simulink model "SIMULATION FILE"  (R2023b)
settings: Solver=VariableStepAuto  StartTime=0.0  StopTime=2.5  RelTol=1e-3
InitFcn:
  | Rs1=0.22;
  | Rsh1=100000;
  | Voc1=0.7;
  | Isc1=0.04;
  | 
  | Rs2=0.22;
  | Rsh2=360;
  | Voc2=0.7;
  | Isc2=0.04;
  | 
  | ki=0.00005926;
  | %ki=0;
  | q=1.6e-19;
  | K=1.30e-23;
  | n=1.3;
  | Ego=1.1;
  | Tn=298;
  | Ns=1;
libraries: simulink x2
settings Model: Creator=smdm6  LastModifiedBy=yasaswini

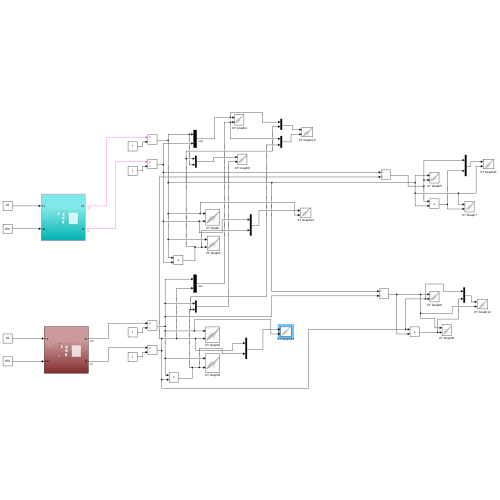
[thumbnail: Simulink's stored preview of the top-level diagram]
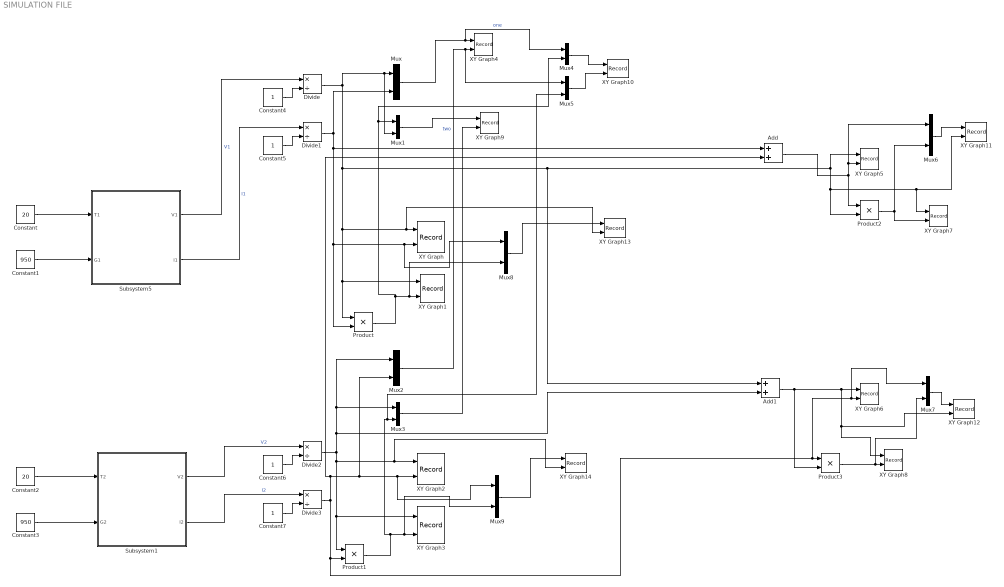
== system SIMULATION FILE ==
  Add : Sum
  Add1 : Sum
  Constant : Constant  Value=20
  Constant1 : Constant  Value=950
  Constant2 : Constant  Value=20
  Constant3 : Constant  Value=950
  Constant{4..7} (4 alike) : Constant
  Divide{,1..3} (4 alike) : Product  Inputs=*/
  Mux{,1..9} (10 alike) : Mux  Inputs=2
  Product{,1..3} (4 alike) : Product
  Subsystem1 : Subsystem
  Subsystem5 : Subsystem
  XY Graph : Record  FileSettingsInternal="{\"entries\":[{\"content\":{\"excelSettings\":{\"content\":{},\"type\":\"Streamout.ExcelSettings\"}},\"type\":\"Streamout.FileSettingStorage\",\"uuid\":\"\"}],\"packageUris\":[\"http:\\/\\/schema.mathworks.com\\/mf0\\/streamout_blocks\\/R2020a\"],\"version\":\"1.0\"}"  Layout=[1 1]  SignalsInternal="{\"entries\":[{\"content\":{\"signals\":[{\"content\":{\"blockPath\":[],\"dimensions\":[1],\"domain\":\"\",\"lineColor\":\"#edb120\",\"port\":1,\"sid\":[\"\"],\"signalID\":1,\"signalName\":\"Divide\"},\"type\":\"RecordBlkView.Signal\",\"uuid\":\"\"},{\"content\":{\"blockPath\":[],\"dimensions\":[1],\"domain\":\"\",\"lineColor\":\"#7e2f8e\",\"port\":2,\"sid\":[\"\"],\"signalID\":2,\"signalName\":\"Divide1\"},\"type\":\"RecordBlkView.Signal\",\"uuid\":\"\"}]},\"type\":\"RecordBlkView.InputSignals\",\"uuid\":\"\"}],\"packageUris\":[\"http:\\/\\/schema.mathworks.com\\/mf0\\/streamout_blocks\\/R2020a\"],\"version\":\"1.0\"}"  VisualizationBindings="{\"xyplotplugin\":{\"info\":[{\"series\":[],\"subplotID\":1}]}}"  CompatibilityTag=XY  st=-1
  XY Graph1 : Record  FileSettingsInternal="{\"entries\":[{\"content\":{\"excelSettings\":{\"content\":{},\"type\":\"Streamout.ExcelSettings\"}},\"type\":\"Streamout.FileSettingStorage\",\"uuid\":\"\"}],\"packageUris\":[\"http:\\/\\/schema.mathworks.com\\/mf0\\/streamout_blocks\\/R2020a\"],\"version\":\"1.0\"}"  Layout=[1 1]  SignalsInternal="{\"entries\":[{\"content\":{\"signals\":[{\"content\":{\"blockPath\":[],\"dimensions\":[1],\"domain\":\"\",\"lineColor\":\"#77ac30\",\"port\":1,\"sid\":[\"\"],\"signalID\":1,\"signalName\":\"Divide\"},\"type\":\"RecordBlkView.Signal\",\"uuid\":\"\"},{\"content\":{\"blockPath\":[],\"dimensions\":[1],\"domain\":\"\",\"lineColor\":\"#4dbeee\",\"port\":2,\"sid\":[\"\"],\"signalID\":2,\"signalName\":\"Product\"},\"type\":\"RecordBlkView.Signal\",\"uuid\":\"\"}]},\"type\":\"RecordBlkView.InputSignals\",\"uuid\":\"\"}],\"packageUris\":[\"http:\\/\\/schema.mathworks.com\\/mf0\\/streamout_blocks\\/R2020a\"],\"version\":\"1.0\"}"  VisualizationBindings="{\"xyplotplugin\":{\"info\":[{\"series\":[],\"subplotID\":1}]}}"  CompatibilityTag=XY  st=-1
  XY Graph10 : Record  FileSettingsInternal="{\"entries\":[{\"content\":{\"excelSettings\":{\"content\":{},\"type\":\"Streamout.ExcelSettings\"}},\"type\":\"Streamout.FileSettingStorage\",\"uuid\":\"\"}],\"packageUris\":[\"http:\\/\\/schema.mathworks.com\\/mf0\\/streamout_blocks\\/R2020a\"],\"version\":\"1.0\"}"  Layout=[1 1]  SignalsInternal="{\"entries\":[{\"content\":{\"signals\":[{\"content\":{\"blockPath\":[],\"dimensions\":[3],\"domain\":\"\",\"hasChildren\":true,\"lineColor\":\"#a2142f\",\"port\":1,\"sid\":[\"\"],\"signalID\":1,\"signalName\":\"Mux4\"},\"type\":\"RecordBlkView.Signal\",\"uuid\":\"\"},{\"content\":{\"blockPath\":[],\"channel\":[1],\"dimensions\":[3],\"domain\":\"\",\"lineColor\":\"#139fff\",\"parentID\":1,\"port\":1,\"sid\":[\"\"],\"signalID\":2,\"signalName\":\"Mux4\"},\"type\":\"RecordBlkView.Signal\",\"uuid\":\"\"},{\"content\":{\"blockPath\":[],\"dimensions\":[3],\"domain\":\"\",\"hasChildren\":true,\"lineColor\":\"#ff6929\",\"port\":2,\"sid\":[\"\"],\"signalID\":3,\"signalName\":\"Mux5\"},\"type\":\"RecordBlkView.Signal\",\"uuid\":\"\"},{\"content\":{\"blockPath\":[],\"channel\":[1],\"dimensions\":[3],\"domain\":\"\",\"lineColor\":\"#b746ff\",\"parentID\":3,\"port\":2,\"sid\":[\"\"],\"signalID\":4,\"signalName\":\"Mux5\"},\"type\":\"RecordBlkView.Signal\",\"uuid\":\"\"},{\"content\":{\"blockPath\":[],\"channel\":[2],\"dimensions\":[3],\"domain\":\"\",\"lineColor\":\"#0072bd\",\"parentID\":1,\"port\":1,\"sid\":[\"\"],\"signalID\":5,\"signalName\":\"Mux4\"},\"type\":\"RecordBlkView.Signal\",\"uuid\":\"\"},{\"content\":{\"blockPath\":[],\"channel\":[3],\"dimensions\":[3],\"domain\":\"\",\"lineColor\":\"#d95319\",\"parentID\":1,\"port\":1,\"sid\":[\"\"],\"signalID\":6,\"signalName\":\"Mux4\"},\"type\":\"RecordBlkView.Signal\",\"uuid\":\"\"},{\"content\":{\"blockPath\":[],\"channel\":[2],\"dimensions\":[3],\"domain\":\"\",\"lineColor\":\"#edb120\",\"parentID\":3,\"port\":2,\"sid\":[\"\"],\"signalID\":7,\"signalName\":\"Mux5\"},\"type\":\"RecordBlkView.Signal\",\"uuid\":\"\"},{\"content\":{\"blockPath\":[],\"channel\":[3],\"dimensions\":[3],\"domain\":\"\",\"lineColor\":\"#7e2f8e\",\"parentID\":3,\"port\":2,\"sid\":[\"\"],\"signalID\":8,\"signalName\":\"Mux5\"},\"type\":\"RecordBlkView.Signal\",\"uuid\":\"\"}]},\"type\":\"RecordBlkView.InputSignals\",\"uuid\":\"\"}],\"packageUris\":[\"http:\\/\\/schema.mathworks.com\\/mf0\\/streamout_blocks\\/R2020a\"],\"version\":\"1.0\"}"  VisualizationBindings="{\"xyplotplugin\":{\"info\":[{\"series\":[],\"subplotID\":1}]}}"  CompatibilityTag=XY
  XY Graph11 : Record  FileSettingsInternal="{\"entries\":[{\"content\":{\"excelSettings\":{\"content\":{},\"type\":\"Streamout.ExcelSettings\"}},\"type\":\"Streamout.FileSettingStorage\",\"uuid\":\"\"}],\"packageUris\":[\"http:\\/\\/schema.mathworks.com\\/mf0\\/streamout_blocks\\/R2020a\"],\"version\":\"1.0\"}"  Layout=[1 1]  SignalsInternal="{\"entries\":[{\"content\":{\"signals\":[{\"content\":{\"blockPath\":[],\"dimensions\":[2],\"domain\":\"\",\"hasChildren\":true,\"lineColor\":\"#64d413\",\"port\":1,\"sid\":[\"\"],\"signalID\":1,\"signalName\":\"Mux6\"},\"type\":\"RecordBlkView.Signal\",\"uuid\":\"\"},{\"content\":{\"blockPath\":[],\"channel\":[1],\"dimensions\":[2],\"domain\":\"\",\"lineColor\":\"#ff13a6\",\"parentID\":1,\"port\":1,\"sid\":[\"\"],\"signalID\":2,\"signalName\":\"Mux6\"},\"type\":\"RecordBlkView.Signal\",\"uuid\":\"\"},{\"content\":{\"blockPath\":[],\"dimensions\":[1],\"domain\":\"\",\"lineColor\":\"#fe330a\",\"port\":2,\"sid\":[\"\"],\"signalID\":3,\"signalName\":\"Divide\"},\"type\":\"RecordBlkView.Signal\",\"uuid\":\"\"},{\"content\":{\"blockPath\":[],\"channel\":[2],\"dimensions\":[2],\"domain\":\"\",\"lineColor\":\"#77ac30\",\"parentID\":1,\"port\":1,\"sid\":[\"\"],\"signalID\":4,\"signalName\":\"Mux6\"},\"type\":\"RecordBlkView.Signal\",\"uuid\":\"\"}]},\"type\":\"RecordBlkView.InputSignals\",\"uuid\":\"\"}],\"packageUris\":[\"http:\\/\\/schema.mathworks.com\\/mf0\\/streamout_blocks\\/R2020a\"],\"version\":\"1.0\"}"  VisualizationBindings="{\"xyplotplugin\":{\"info\":[{\"series\":[],\"subplotID\":1}]}}"  CompatibilityTag=XY
  XY Graph12 : Record  FileSettingsInternal="{\"entries\":[{\"content\":{\"excelSettings\":{\"content\":{},\"type\":\"Streamout.ExcelSettings\"}},\"type\":\"Streamout.FileSettingStorage\",\"uuid\":\"\"}],\"packageUris\":[\"http:\\/\\/schema.mathworks.com\\/mf0\\/streamout_blocks\\/R2020a\"],\"version\":\"1.0\"}"  Layout=[1 1]  SignalsInternal="{\"entries\":[{\"content\":{\"signals\":[{\"content\":{\"blockPath\":[],\"dimensions\":[2],\"domain\":\"\",\"hasChildren\":true,\"lineColor\":\"#22b573\",\"port\":1,\"sid\":[\"\"],\"signalID\":1,\"signalName\":\"Mux7\"},\"type\":\"RecordBlkView.Signal\",\"uuid\":\"\"},{\"content\":{\"blockPath\":[],\"channel\":[1],\"dimensions\":[2],\"domain\":\"\",\"lineColor\":\"#0072bd\",\"parentID\":1,\"port\":1,\"sid\":[\"\"],\"signalID\":2,\"signalName\":\"Mux7\"},\"type\":\"RecordBlkView.Signal\",\"uuid\":\"\"},{\"content\":{\"blockPath\":[],\"dimensions\":[1],\"domain\":\"\",\"lineColor\":\"#d95319\",\"port\":2,\"sid\":[\"\"],\"signalID\":3,\"signalName\":\"Add1\"},\"type\":\"RecordBlkView.Signal\",\"uuid\":\"\"},{\"content\":{\"blockPath\":[],\"channel\":[2],\"dimensions\":[2],\"domain\":\"\",\"lineColor\":\"#4dbeee\",\"parentID\":1,\"port\":1,\"sid\":[\"\"],\"signalID\":4,\"signalName\":\"Mux7\"},\"type\":\"RecordBlkView.Signal\",\"uuid\":\"\"}]},\"type\":\"RecordBlkView.InputSignals\",\"uuid\":\"\"}],\"packageUris\":[\"http:\\/\\/schema.mathworks.com\\/mf0\\/streamout_blocks\\/R2020a\"],\"version\":\"1.0\"}"  VisualizationBindings="{\"xyplotplugin\":{\"info\":[{\"series\":[],\"subplotID\":1}]}}"  CompatibilityTag=XY
  XY Graph13 : Record  FileSettingsInternal="{\"entries\":[{\"content\":{\"excelSettings\":{\"content\":{},\"type\":\"Streamout.ExcelSettings\"}},\"type\":\"Streamout.FileSettingStorage\",\"uuid\":\"\"}],\"packageUris\":[\"http:\\/\\/schema.mathworks.com\\/mf0\\/streamout_blocks\\/R2020a\"],\"version\":\"1.0\"}"  Layout=[1 1]  SignalsInternal="{\"entries\":[{\"content\":{\"signals\":[{\"content\":{\"blockPath\":[],\"dimensions\":[2],\"domain\":\"\",\"hasChildren\":true,\"lineColor\":\"#edb120\",\"port\":1,\"sid\":[\"\"],\"signalID\":1,\"signalName\":\"Mux8\"},\"type\":\"RecordBlkView.Signal\",\"uuid\":\"\"},{\"content\":{\"blockPath\":[],\"channel\":[1],\"dimensions\":[2],\"domain\":\"\",\"lineColor\":\"#7e2f8e\",\"parentID\":1,\"port\":1,\"sid\":[\"\"],\"signalID\":2,\"signalName\":\"Mux8\"},\"type\":\"RecordBlkView.Signal\",\"uuid\":\"\"},{\"content\":{\"blockPath\":[],\"dimensions\":[1],\"domain\":\"\",\"lineColor\":\"#77ac30\",\"port\":2,\"sid\":[\"\"],\"signalID\":3,\"signalName\":\"Divide\"},\"type\":\"RecordBlkView.Signal\",\"uuid\":\"\"},{\"content\":{\"blockPath\":[],\"channel\":[2],\"dimensions\":[2],\"domain\":\"\",\"lineColor\":\"#a2142f\",\"parentID\":1,\"port\":1,\"sid\":[\"\"],\"signalID\":4,\"signalName\":\"Mux8\"},\"type\":\"RecordBlkView.Signal\",\"uuid\":\"\"}]},\"type\":\"RecordBlkView.InputSignals\",\"uuid\":\"\"}],\"packageUris\":[\"http:\\/\\/schema.mathworks.com\\/mf0\\/streamout_blocks\\/R2020a\"],\"version\":\"1.0\"}"  VisualizationBindings="{\"xyplotplugin\":{\"info\":[{\"series\":[],\"subplotID\":1}]}}"  CompatibilityTag=XY
  XY Graph14 : Record  FileSettingsInternal="{\"entries\":[{\"content\":{\"excelSettings\":{\"content\":{},\"type\":\"Streamout.ExcelSettings\"}},\"type\":\"Streamout.FileSettingStorage\",\"uuid\":\"\"}],\"packageUris\":[\"http:\\/\\/schema.mathworks.com\\/mf0\\/streamout_blocks\\/R2020a\"],\"version\":\"1.0\"}"  Layout=[1 1]  SignalsInternal="{\"entries\":[{\"content\":{\"signals\":[{\"content\":{\"blockPath\":[],\"dimensions\":[2],\"domain\":\"\",\"hasChildren\":true,\"lineColor\":\"#4dbeee\",\"port\":1,\"sid\":[\"\"],\"signalID\":1,\"signalName\":\"Mux9\"},\"type\":\"RecordBlkView.Signal\",\"uuid\":\"\"},{\"content\":{\"blockPath\":[],\"channel\":[1],\"dimensions\":[2],\"domain\":\"\",\"lineColor\":\"#a2142f\",\"parentID\":1,\"port\":1,\"sid\":[\"\"],\"signalID\":2,\"signalName\":\"Mux9\"},\"type\":\"RecordBlkView.Signal\",\"uuid\":\"\"},{\"content\":{\"blockPath\":[],\"dimensions\":[1],\"domain\":\"\",\"lineColor\":\"#139fff\",\"port\":2,\"sid\":[\"\"],\"signalID\":3,\"signalName\":\"Divide2\"},\"type\":\"RecordBlkView.Signal\",\"uuid\":\"\"},{\"content\":{\"blockPath\":[],\"channel\":[2],\"dimensions\":[2],\"domain\":\"\",\"lineColor\":\"#139fff\",\"parentID\":1,\"port\":1,\"sid\":[\"\"],\"signalID\":4,\"signalName\":\"Mux9\"},\"type\":\"RecordBlkView.Signal\",\"uuid\":\"\"}]},\"type\":\"RecordBlkView.InputSignals\",\"uuid\":\"\"}],\"packageUris\":[\"http:\\/\\/schema.mathworks.com\\/mf0\\/streamout_blocks\\/R2020a\"],\"version\":\"1.0\"}"  VisualizationBindings="{\"xyplotplugin\":{\"info\":[{\"series\":[],\"subplotID\":1}]}}"  CompatibilityTag=XY
  XY Graph2 : Record  FileSettingsInternal="{\"entries\":[{\"content\":{\"excelSettings\":{\"content\":{},\"type\":\"Streamout.ExcelSettings\"}},\"type\":\"Streamout.FileSettingStorage\",\"uuid\":\"\"}],\"packageUris\":[\"http:\\/\\/schema.mathworks.com\\/mf0\\/streamout_blocks\\/R2020a\"],\"version\":\"1.0\"}"  Layout=[1 1]  SignalsInternal="{\"entries\":[{\"content\":{\"signals\":[{\"content\":{\"blockPath\":[],\"dimensions\":[1],\"domain\":\"\",\"lineColor\":\"#ff6929\",\"port\":1,\"sid\":[\"\"],\"signalID\":1,\"signalName\":\"Divide2\"},\"type\":\"RecordBlkView.Signal\",\"uuid\":\"\"},{\"content\":{\"blockPath\":[],\"dimensions\":[1],\"domain\":\"\",\"lineColor\":\"#b746ff\",\"port\":2,\"sid\":[\"\"],\"signalID\":2,\"signalName\":\"Divide3\"},\"type\":\"RecordBlkView.Signal\",\"uuid\":\"\"}]},\"type\":\"RecordBlkView.InputSignals\",\"uuid\":\"\"}],\"packageUris\":[\"http:\\/\\/schema.mathworks.com\\/mf0\\/streamout_blocks\\/R2020a\"],\"version\":\"1.0\"}"  VisualizationBindings="{\"xyplotplugin\":{\"info\":[{\"series\":[],\"subplotID\":1}]}}"  CompatibilityTag=XY  st=-1
  XY Graph3 : Record  FileSettingsInternal="{\"entries\":[{\"content\":{\"excelSettings\":{\"content\":{},\"type\":\"Streamout.ExcelSettings\"}},\"type\":\"Streamout.FileSettingStorage\",\"uuid\":\"\"}],\"packageUris\":[\"http:\\/\\/schema.mathworks.com\\/mf0\\/streamout_blocks\\/R2020a\"],\"version\":\"1.0\"}"  Layout=[1 1]  SignalsInternal="{\"entries\":[{\"content\":{\"signals\":[{\"content\":{\"blockPath\":[],\"dimensions\":[1],\"domain\":\"\",\"lineColor\":\"#64d413\",\"port\":1,\"sid\":[\"\"],\"signalID\":1,\"signalName\":\"Divide2\"},\"type\":\"RecordBlkView.Signal\",\"uuid\":\"\"},{\"content\":{\"blockPath\":[],\"dimensions\":[1],\"domain\":\"\",\"lineColor\":\"#ff13a6\",\"port\":2,\"sid\":[\"\"],\"signalID\":2,\"signalName\":\"Product1\"},\"type\":\"RecordBlkView.Signal\",\"uuid\":\"\"}]},\"type\":\"RecordBlkView.InputSignals\",\"uuid\":\"\"}],\"packageUris\":[\"http:\\/\\/schema.mathworks.com\\/mf0\\/streamout_blocks\\/R2020a\"],\"version\":\"1.0\"}"  VisualizationBindings="{\"xyplotplugin\":{\"info\":[{\"series\":[],\"subplotID\":1}]}}"  CompatibilityTag=XY  st=-1
  XY Graph4 : Record  FileSettingsInternal="{\"entries\":[{\"content\":{\"excelSettings\":{\"content\":{},\"type\":\"Streamout.ExcelSettings\"}},\"type\":\"Streamout.FileSettingStorage\",\"uuid\":\"\"}],\"packageUris\":[\"http:\\/\\/schema.mathworks.com\\/mf0\\/streamout_blocks\\/R2020a\"],\"version\":\"1.0\"}"  Layout=[1 1]  SignalsInternal="{\"entries\":[{\"content\":{\"signals\":[{\"content\":{\"blockPath\":[],\"dimensions\":[2],\"domain\":\"\",\"hasChildren\":true,\"lineColor\":\"#fe330a\",\"port\":1,\"sid\":[\"\"],\"signalID\":1,\"signalName\":\"one\"},\"type\":\"RecordBlkView.Signal\",\"uuid\":\"\"},{\"content\":{\"blockPath\":[],\"channel\":[1],\"dimensions\":[2],\"domain\":\"\",\"lineColor\":\"#22b573\",\"parentID\":1,\"port\":1,\"sid\":[\"\"],\"signalID\":2,\"signalName\":\"one\"},\"type\":\"RecordBlkView.Signal\",\"uuid\":\"\"},{\"content\":{\"blockPath\":[],\"dimensions\":[2],\"domain\":\"\",\"hasChildren\":true,\"lineColor\":\"#0072bd\",\"port\":2,\"sid\":[\"\"],\"signalID\":3,\"signalName\":\"two\"},\"type\":\"RecordBlkView.Signal\",\"uuid\":\"\"},{\"content\":{\"blockPath\":[],\"channel\":[1],\"dimensions\":[2],\"domain\":\"\",\"lineColor\":\"#d95319\",\"parentID\":3,\"port\":2,\"sid\":[\"\"],\"signalID\":4,\"signalName\":\"two\"},\"type\":\"RecordBlkView.Signal\",\"uuid\":\"\"},{\"content\":{\"blockPath\":[],\"channel\":[2],\"dimensions\":[2],\"domain\":\"\",\"lineColor\":\"#ff6929\",\"parentID\":1,\"port\":1,\"sid\":[\"\"],\"signalID\":5,\"signalName\":\"one\"},\"type\":\"RecordBlkView.Signal\",\"uuid\":\"\"},{\"content\":{\"blockPath\":[],\"channel\":[2],\"dimensions\":[2],\"domain\":\"\",\"lineColor\":\"#b746ff\",\"parentID\":3,\"port\":2,\"sid\":[\"\"],\"signalID\":6,\"signalName\":\"two\"},\"type\":\"RecordBlkView.Signal\",\"uuid\":\"\"}]},\"type\":\"RecordBlkView.InputSignals\",\"uuid\":\"\"}],\"packageUris\":[\"http:\\/\\/schema.mathworks.com\\/mf0\\/streamout_blocks\\/R2020a\"],\"version\":\"1.0\"}"  VisualizationBindings="{\"xyplotplugin\":{\"info\":[{\"series\":[],\"subplotID\":1}]}}"  CompatibilityTag=XY  st=-1
  XY Graph5 : Record  FileSettingsInternal="{\"entries\":[{\"content\":{\"excelSettings\":{\"content\":{},\"type\":\"Streamout.ExcelSettings\"}},\"type\":\"Streamout.FileSettingStorage\",\"uuid\":\"\"}],\"packageUris\":[\"http:\\/\\/schema.mathworks.com\\/mf0\\/streamout_blocks\\/R2020a\"],\"version\":\"1.0\"}"  Layout=[1 1]  SignalsInternal="{\"entries\":[{\"content\":{\"signals\":[{\"content\":{\"blockPath\":[],\"dimensions\":[1],\"domain\":\"\",\"lineColor\":\"#edb120\",\"port\":1,\"sid\":[\"\"],\"signalID\":1,\"signalName\":\"Divide\"},\"type\":\"RecordBlkView.Signal\",\"uuid\":\"\"},{\"content\":{\"blockPath\":[],\"dimensions\":[1],\"domain\":\"\",\"lineColor\":\"#7e2f8e\",\"port\":2,\"sid\":[\"\"],\"signalID\":2,\"signalName\":\"Add\"},\"type\":\"RecordBlkView.Signal\",\"uuid\":\"\"}]},\"type\":\"RecordBlkView.InputSignals\",\"uuid\":\"\"}],\"packageUris\":[\"http:\\/\\/schema.mathworks.com\\/mf0\\/streamout_blocks\\/R2020a\"],\"version\":\"1.0\"}"  VisualizationBindings="{\"xyplotplugin\":{\"info\":[{\"series\":[],\"subplotID\":1}]}}"  CompatibilityTag=XY  st=-1
  XY Graph6 : Record  FileSettingsInternal="{\"entries\":[{\"content\":{\"excelSettings\":{\"content\":{},\"type\":\"Streamout.ExcelSettings\"}},\"type\":\"Streamout.FileSettingStorage\",\"uuid\":\"\"}],\"packageUris\":[\"http:\\/\\/schema.mathworks.com\\/mf0\\/streamout_blocks\\/R2020a\"],\"version\":\"1.0\"}"  Layout=[1 1]  SignalsInternal="{\"entries\":[{\"content\":{\"signals\":[{\"content\":{\"blockPath\":[],\"dimensions\":[1],\"domain\":\"\",\"lineColor\":\"#77ac30\",\"port\":1,\"sid\":[\"\"],\"signalID\":1,\"signalName\":\"Add1\"},\"type\":\"RecordBlkView.Signal\",\"uuid\":\"\"},{\"content\":{\"blockPath\":[],\"dimensions\":[1],\"domain\":\"\",\"lineColor\":\"#4dbeee\",\"port\":2,\"sid\":[\"\"],\"signalID\":2,\"signalName\":\"Divide3\"},\"type\":\"RecordBlkView.Signal\",\"uuid\":\"\"}]},\"type\":\"RecordBlkView.InputSignals\",\"uuid\":\"\"}],\"packageUris\":[\"http:\\/\\/schema.mathworks.com\\/mf0\\/streamout_blocks\\/R2020a\"],\"version\":\"1.0\"}"  VisualizationBindings="{\"xyplotplugin\":{\"info\":[{\"series\":[],\"subplotID\":1}]}}"  CompatibilityTag=XY  st=-1
  XY Graph7 : Record  FileSettingsInternal="{\"entries\":[{\"content\":{\"excelSettings\":{\"content\":{},\"type\":\"Streamout.ExcelSettings\"}},\"type\":\"Streamout.FileSettingStorage\",\"uuid\":\"\"}],\"packageUris\":[\"http:\\/\\/schema.mathworks.com\\/mf0\\/streamout_blocks\\/R2020a\"],\"version\":\"1.0\"}"  Layout=[1 1]  SignalsInternal="{\"entries\":[{\"content\":{\"signals\":[{\"content\":{\"blockPath\":[],\"dimensions\":[1],\"domain\":\"\",\"lineColor\":\"#a2142f\",\"port\":1,\"sid\":[\"\"],\"signalID\":1,\"signalName\":\"Divide\"},\"type\":\"RecordBlkView.Signal\",\"uuid\":\"\"},{\"content\":{\"blockPath\":[],\"dimensions\":[1],\"domain\":\"\",\"lineColor\":\"#139fff\",\"port\":2,\"sid\":[\"\"],\"signalID\":2,\"signalName\":\"Product2\"},\"type\":\"RecordBlkView.Signal\",\"uuid\":\"\"}]},\"type\":\"RecordBlkView.InputSignals\",\"uuid\":\"\"}],\"packageUris\":[\"http:\\/\\/schema.mathworks.com\\/mf0\\/streamout_blocks\\/R2020a\"],\"version\":\"1.0\"}"  VisualizationBindings="{\"xyplotplugin\":{\"info\":[{\"series\":[],\"subplotID\":1}]}}"  CompatibilityTag=XY  st=-1
  XY Graph8 : Record  FileSettingsInternal="{\"entries\":[{\"content\":{\"excelSettings\":{\"content\":{},\"type\":\"Streamout.ExcelSettings\"}},\"type\":\"Streamout.FileSettingStorage\",\"uuid\":\"\"}],\"packageUris\":[\"http:\\/\\/schema.mathworks.com\\/mf0\\/streamout_blocks\\/R2020a\"],\"version\":\"1.0\"}"  Layout=[1 1]  SignalsInternal="{\"entries\":[{\"content\":{\"signals\":[{\"content\":{\"blockPath\":[],\"dimensions\":[1],\"domain\":\"\",\"lineColor\":\"#ff6929\",\"port\":1,\"sid\":[\"\"],\"signalID\":1,\"signalName\":\"Add1\"},\"type\":\"RecordBlkView.Signal\",\"uuid\":\"\"},{\"content\":{\"blockPath\":[],\"dimensions\":[1],\"domain\":\"\",\"lineColor\":\"#b746ff\",\"port\":2,\"sid\":[\"\"],\"signalID\":2,\"signalName\":\"Product3\"},\"type\":\"RecordBlkView.Signal\",\"uuid\":\"\"}]},\"type\":\"RecordBlkView.InputSignals\",\"uuid\":\"\"}],\"packageUris\":[\"http:\\/\\/schema.mathworks.com\\/mf0\\/streamout_blocks\\/R2020a\"],\"version\":\"1.0\"}"  VisualizationBindings="{\"xyplotplugin\":{\"info\":[{\"series\":[],\"subplotID\":1}]}}"  CompatibilityTag=XY  st=-1
  XY Graph9 : Record  FileSettingsInternal="{\"entries\":[{\"content\":{\"excelSettings\":{\"content\":{},\"type\":\"Streamout.ExcelSettings\"}},\"type\":\"Streamout.FileSettingStorage\",\"uuid\":\"\"}],\"packageUris\":[\"http:\\/\\/schema.mathworks.com\\/mf0\\/streamout_blocks\\/R2020a\"],\"version\":\"1.0\"}"  Layout=[1 1]  SignalsInternal="{\"entries\":[{\"content\":{\"signals\":[{\"content\":{\"blockPath\":[],\"dimensions\":[2],\"domain\":\"\",\"hasChildren\":true,\"lineColor\":\"#64d413\",\"port\":1,\"sid\":[\"\"],\"signalID\":1,\"signalName\":\"Mux1\"},\"type\":\"RecordBlkView.Signal\",\"uuid\":\"\"},{\"content\":{\"blockPath\":[],\"channel\":[1],\"dimensions\":[2],\"domain\":\"\",\"lineColor\":\"#ff13a6\",\"parentID\":1,\"plots\":[ 1 ],\"port\":1,\"sid\":[\"\"],\"signalID\":2,\"signalName\":\"Mux1\"},\"type\":\"RecordBlkView.Signal\",\"uuid\":\"\"},{\"content\":{\"blockPath\":[],\"dimensions\":[2],\"domain\":\"\",\"hasChildren\":true,\"lineColor\":\"#fe330a\",\"port\":2,\"sid\":[\"\"],\"signalID\":3,\"signalName\":\"Mux3\"},\"type\":\"RecordBlkView.Signal\",\"uuid\":\"\"},{\"content\":{\"blockPath\":[],\"channel\":[1],\"dimensions\":[2],\"domain\":\"\",\"lineColor\":\"#22b573\",\"parentID\":3,\"plots\":[ 1 ],\"port\":2,\"sid\":[\"\"],\"signalID\":4,\"signalName\":\"Mux3\"},\"type\":\"RecordBlkView.Signal\",\"uuid\":\"\"},{\"content\":{\"blockPath\":[],\"channel\":[2],\"dimensions\":[2],\"domain\":\"\",\"lineColor\":\"#edb120\",\"parentID\":1,\"plots\":[ 1 ],\"port\":1,\"sid\":[\"\"],\"signalID\":5,\"signalName\":\"Mux1\"},\"type\":\"RecordBlkView.Signal\",\"uuid\":\"\"},{\"content\":{\"blockPath\":[],\"channel\":[2],\"dimensions\":[2],\"domain\":\"\",\"lineColor\":\"#7e2f8e\",\"parentID\":3,\"plots\":[ 1 ],\"port\":2,\"sid\":[\"\"],\"signalID\":6,\"signalName\":\"Mux3\"},\"type\":\"RecordBlkView.Signal\",\"uuid\":\"\"}]},\"type\":\"RecordBlkView.InputSignals\",\"uuid\":\"\"}],\"packageUris\":[\"http:\\/\\/schema.mathworks.com\\/mf0\\/streamout_blocks\\/R2020a\"],\"version\":\"1.0\"}"  VisualizationBindings="{\"xyplotplugin\":{\"info\":[{\"series\":[{\"bindingParametersList\":[{\"parameter\":\"X-Axis\",\"signalID\":5,\"signalName\":\"Mux1(2)\"},{\"parameter\":\"Y-Axis\",\"signalID\":2,\"signalName\":\"Mux1(1)\"}],\"seriesID\":0},{\"bindingParametersList\":[{\"parameter\":\"X-Axis\",\"signalID\":4,\"signalName\":\"Mux3(1)\"},{\"parameter\":\"Y-Axis\",\"signalID\":6,\"signalName\":\"Mux3(2)\"}],\"seriesID\":1}],\"subplotID\":1}]}}"  CompatibilityTag=XY  st=-1
  wires:
  Mux2/1 -> Mux5/1, XY Graph4/2  "two"
  Divide/1 -> Mux1/2, Mux/1, Product2/2, XY Graph11/2, XY Graph7/1, XY Graph5/1, Add1/1, XY Graph13/2, XY Graph/1, XY Graph1/1, Product/1
  Subsystem1/1(V2) -> Divide2/1  "V2"
  Mux3/1 -> XY Graph9/2
  Mux/1 -> Mux4/1, XY Graph4/1  "one"
  Subsystem1/2(I2) -> Divide3/1  "I2"
  Mux1/1 -> XY Graph9/1
  Product/1 -> Mux4/2, Mux1/1, Mux8/2, XY Graph1/2
  Constant6/1 -> Divide2/2
  Product1/1 -> Mux5/2, Mux3/2, Mux9/2, XY Graph3/2
  Divide3/1 -> Mux7/1, XY Graph6/2, Product3/1, Product1/2, Add/2, Mux2/2, Mux9/1, XY Graph2/2
  Divide2/1 -> Mux2/1, Mux3/1, Add1/2, XY Graph14/2, XY Graph2/1, Product1/1, XY Graph3/1
  Divide1/1 -> Mux/2, Add/1, Product/2, Mux8/1, XY Graph/2
  Constant7/1 -> Divide3/2
  Subsystem5/1(V1) -> Divide/1  "V1"
  Subsystem5/2(I1) -> Divide1/1  "I1"
  Constant/1 -> Subsystem5/1(T1)
  Add1/1 -> Product3/2, XY Graph8/1, XY Graph12/2, XY Graph6/1
  Constant2/1 -> Subsystem1/1(T2)
  Constant3/1 -> Subsystem1/2(G2)
  Constant1/1 -> Subsystem5/2(G1)
  Product2/1 -> Mux6/2, XY Graph7/2
  Constant5/1 -> Divide1/2
  Product3/1 -> Mux7/2, XY Graph8/2
  Add/1 -> XY Graph5/2, Mux6/1, Product2/1
  Constant4/1 -> Divide/2
  Mux4/1 -> XY Graph10/1
  Mux5/1 -> XY Graph10/2
  Mux6/1 -> XY Graph11/1
  Mux7/1 -> XY Graph12/1
  Mux8/1 -> XY Graph13/1
  Mux9/1 -> XY Graph14/1

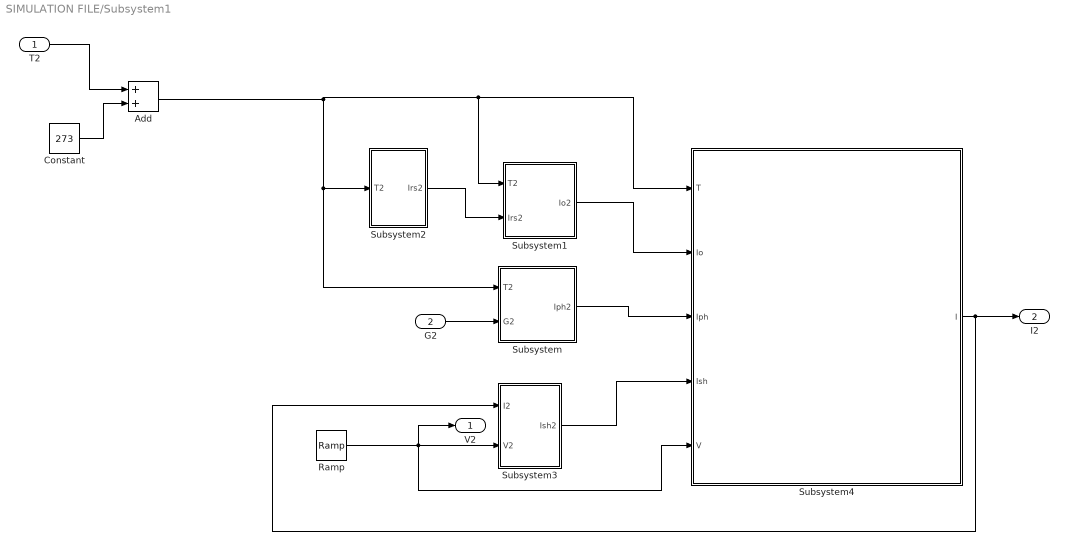
== system SIMULATION FILE/Subsystem1 ==
  T2 : Inport
  G2 : Inport  Port=2
  Add : Sum
  Constant : Constant  Value=273
  Ramp : simulink/Sources/Ramp  slope=0.2187  start=0  InitialOutput=0
  Subsystem : Subsystem
  Subsystem1 : Subsystem
  Subsystem2 : Subsystem
  Subsystem3 : Subsystem
  Subsystem4 : Subsystem
  V2 : Outport
  I2 : Outport  Port=2
  wires:
  Subsystem/1(Iph2) -> Subsystem4/3(Iph)
  G2/1 -> Subsystem/2(G2)
  Constant/1 -> Add/2
  Subsystem2/1(Irs2) -> Subsystem1/2(Irs2)
  Subsystem4/1(I) -> I2/1, Subsystem3/1(I2)
  Add/1 -> Subsystem1/1(T2), Subsystem4/1(T), Subsystem2/1(T2), Subsystem/1(T2)
  Subsystem3/1(Ish2) -> Subsystem4/4(Ish)
  Ramp/1 -> V2/1, Subsystem4/5(V), Subsystem3/2(V2)
  Subsystem1/1(Io2) -> Subsystem4/2(Io)
  T2/1 -> Add/1

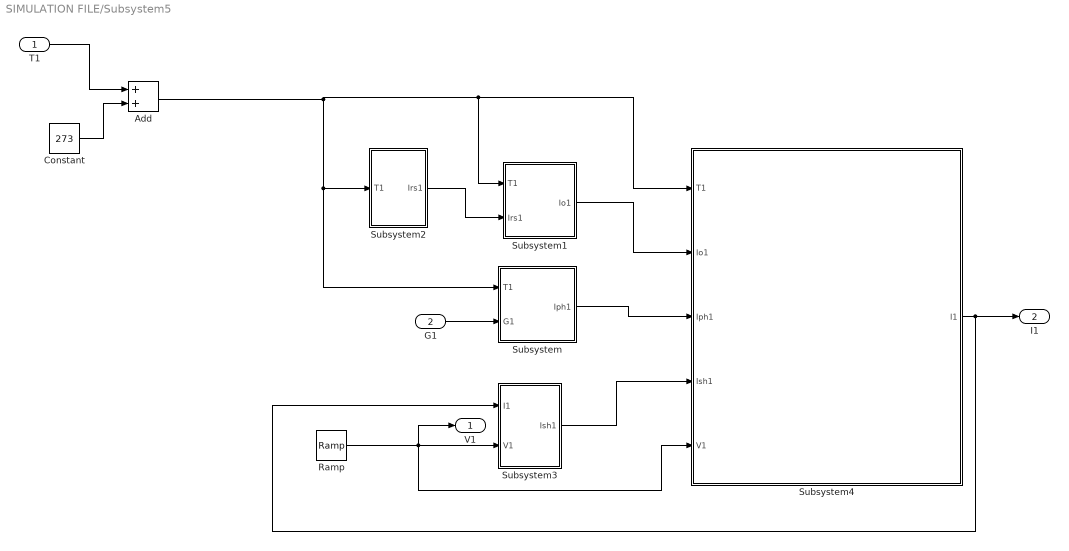
== system SIMULATION FILE/Subsystem5 ==
  T1 : Inport
  G1 : Inport  Port=2
  Add : Sum
  Constant : Constant  Value=273
  Ramp : simulink/Sources/Ramp  slope=0.2187  start=0  InitialOutput=0
  Subsystem : Subsystem
  Subsystem1 : Subsystem
  Subsystem2 : Subsystem
  Subsystem3 : Subsystem
  Subsystem4 : Subsystem
  V1 : Outport
  I1 : Outport  Port=2
  wires:
  Subsystem/1(Iph1) -> Subsystem4/3(Iph1)
  G1/1 -> Subsystem/2(G1)
  Constant/1 -> Add/2
  Subsystem2/1(Irs1) -> Subsystem1/2(Irs1)
  Subsystem4/1(I1) -> I1/1, Subsystem3/1(I1)
  Add/1 -> Subsystem1/1(T1), Subsystem4/1(T1), Subsystem2/1(T1), Subsystem/1(T1)
  Subsystem3/1(Ish1) -> Subsystem4/4(Ish1)
  Ramp/1 -> V1/1, Subsystem4/5(V1), Subsystem3/2(V1)
  Subsystem1/1(Io1) -> Subsystem4/2(Io1)
  T1/1 -> Add/1

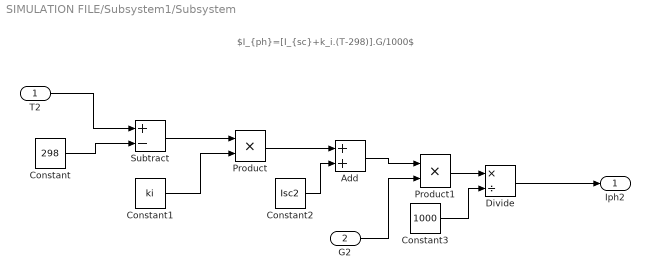
== system SIMULATION FILE/Subsystem1/Subsystem ==
  note: $I_{ph}=[I_{sc}+k_i.(T-298)].G/1000$
  T2 : Inport
  G2 : Inport  Port=2
  Add : Sum
  Constant : Constant  Value=298
  Constant1 : Constant  Value=ki
  Constant2 : Constant  Value=Isc2
  Constant3 : Constant  Value=1000
  Divide : Product  Inputs=*/
  Product : Product
  Product1 : Product
  Subtract : Sum  Inputs=+-
  Iph2 : Outport
  wires:
  G2/1 -> Product1/2
  Constant/1 -> Subtract/2
  T2/1 -> Subtract/1
  Subtract/1 -> Product/1
  Add/1 -> Product1/1
  Constant1/1 -> Product/2
  Product/1 -> Add/1
  Constant2/1 -> Add/2
  Constant3/1 -> Divide/2
  Product1/1 -> Divide/1
  Divide/1 -> Iph2/1

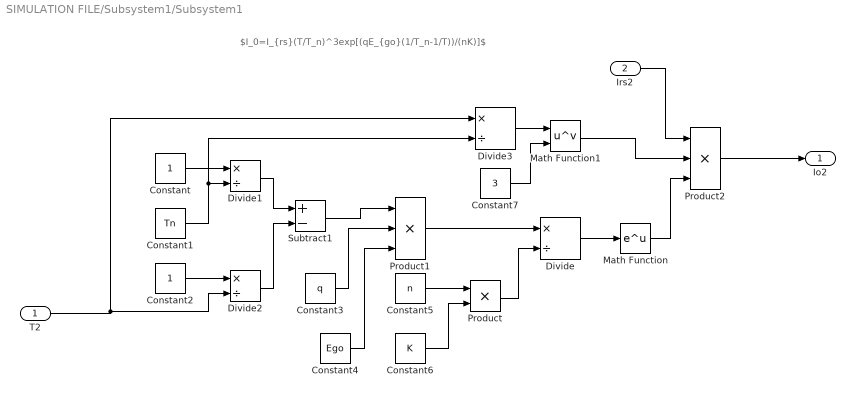
== system SIMULATION FILE/Subsystem1/Subsystem1 ==
  note: $I_0=I_{rs}(T/T_n)^3exp[(qE_{go}(1/T_n-1/T))/(nK)]$
  T2 : Inport
  Irs2 : Inport  Port=2
  Constant : Constant
  Constant1 : Constant  Value=Tn
  Constant2 : Constant
  Constant3 : Constant  Value=q
  Constant4 : Constant  Value=Ego
  Constant5 : Constant  Value=n
  Constant6 : Constant  Value=K
  Constant7 : Constant  Value=3
  Divide{,1..3} (4 alike) : Product  Inputs=*/
  Math Function : Math
  Math Function1 : Math  Operator=pow
  Product : Product
  Product1 : Product  Inputs=3
  Product2 : Product  Inputs=3
  Subtract1 : Sum  Inputs=+-
  Io2 : Outport
  wires:
  Constant6/1 -> Product/2
  Product1/1 -> Divide/1
  Math Function/1 -> Product2/3
  Subtract1/1 -> Product1/1
  Constant2/1 -> Divide2/1
  Divide3/1 -> Math Function1/1
  Divide/1 -> Math Function/1
  Constant7/1 -> Math Function1/2
  Irs2/1 -> Product2/1
  Product/1 -> Divide/2
  Divide1/1 -> Subtract1/1
  Constant5/1 -> Product/1
  Divide2/1 -> Subtract1/2
  T2/1 -> Divide3/1, Divide2/2
  Constant1/1 -> Divide3/2, Divide1/2
  Constant/1 -> Divide1/1
  Constant4/1 -> Product1/3
  Constant3/1 -> Product1/2
  Math Function1/1 -> Product2/2
  Product2/1 -> Io2/1

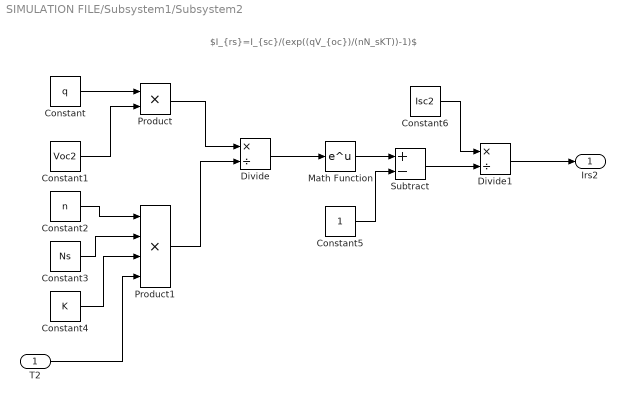
== system SIMULATION FILE/Subsystem1/Subsystem2 ==
  note: $I_{rs}=I_{sc}/(exp((qV_{oc})/(nN_sKT))-1)$
  T2 : Inport
  Constant : Constant  Value=q
  Constant1 : Constant  Value=Voc2
  Constant2 : Constant  Value=n
  Constant3 : Constant  Value=Ns
  Constant4 : Constant  Value=K
  Constant5 : Constant
  Constant6 : Constant  Value=Isc2
  Divide : Product  Inputs=*/
  Divide1 : Product  Inputs=*/
  Math Function : Math
  Product : Product
  Product1 : Product  Inputs=4
  Subtract : Sum  Inputs=+-
  Irs2 : Outport
  wires:
  Constant5/1 -> Subtract/2
  Product/1 -> Divide/1
  Subtract/1 -> Divide1/2
  Math Function/1 -> Subtract/1
  Divide1/1 -> Irs2/1
  Constant2/1 -> Product1/1
  Product1/1 -> Divide/2
  Constant1/1 -> Product/2
  Constant3/1 -> Product1/2
  Divide/1 -> Math Function/1
  Constant4/1 -> Product1/3
  Constant6/1 -> Divide1/1
  Constant/1 -> Product/1
  T2/1 -> Product1/4

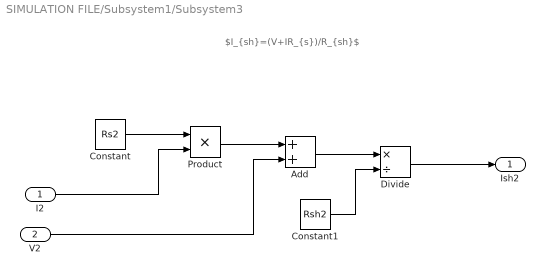
== system SIMULATION FILE/Subsystem1/Subsystem3 ==
  note: $I_{sh}=(V+IR_{s})/R_{sh}$
  I2 : Inport
  V2 : Inport  Port=2
  Add : Sum
  Constant : Constant  Value=Rs2
  Constant1 : Constant  Value=Rsh2
  Divide : Product  Inputs=*/
  Product : Product
  Ish2 : Outport
  wires:
  Constant1/1 -> Divide/2
  Product/1 -> Add/1
  V2/1 -> Add/2
  I2/1 -> Product/2
  Divide/1 -> Ish2/1
  Constant/1 -> Product/1
  Add/1 -> Divide/1

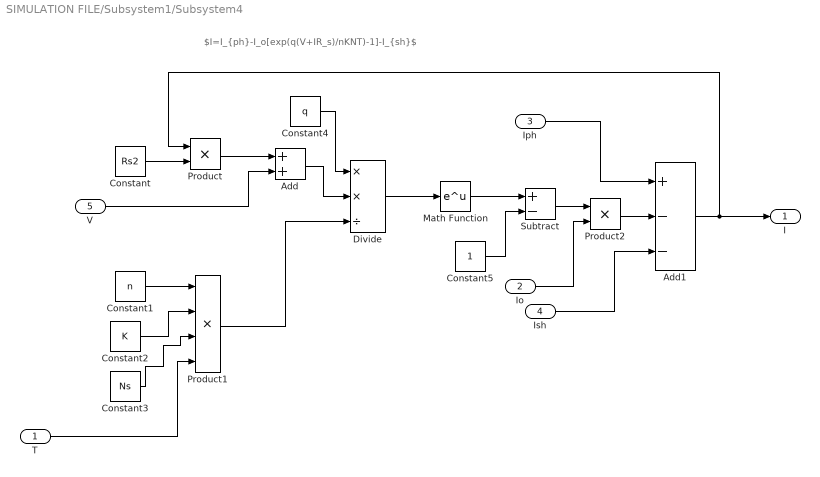
== system SIMULATION FILE/Subsystem1/Subsystem4 ==
  note: $I=I_{ph}-I_o[exp(q(V+IR_s)/nKNT)-1]-I_{sh}$
  T : Inport
  Io : Inport  Port=2
  Iph : Inport  Port=3
  Ish : Inport  Port=4
  V : Inport  Port=5
  Add : Sum
  Add1 : Sum  Inputs=+--
  Constant : Constant  Value=Rs2
  Constant1 : Constant  Value=n
  Constant2 : Constant  Value=K
  Constant3 : Constant  Value=Ns
  Constant4 : Constant  Value=q
  Constant5 : Constant
  Divide : Product  Inputs=**/
  Math Function : Math
  Product : Product
  Product1 : Product  Inputs=4
  Product2 : Product
  Subtract : Sum  Inputs=+-
  I : Outport
  wires:
  Constant3/1 -> Product1/3
  Subtract/1 -> Product2/1
  Constant1/1 -> Product1/1
  Divide/1 -> Math Function/1
  Constant4/1 -> Divide/1
  Product1/1 -> Divide/3
  Constant2/1 -> Product1/2
  Math Function/1 -> Subtract/1
  T/1 -> Product1/4
  Product2/1 -> Add1/2
  Constant/1 -> Product/2
  Product/1 -> Add/1
  Constant5/1 -> Subtract/2
  Add/1 -> Divide/2
  Add1/1 -> I/1, Product/1
  V/1 -> Add/2
  Io/1 -> Product2/2
  Ish/1 -> Add1/3
  Iph/1 -> Add1/1

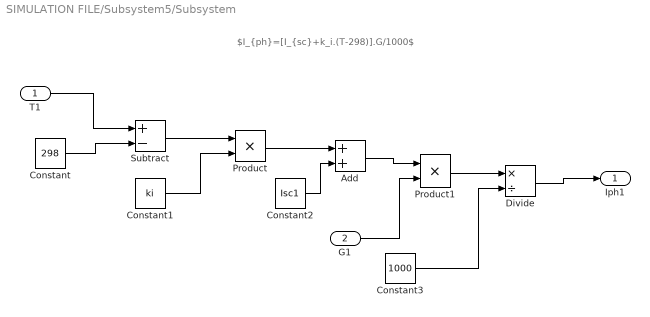
== system SIMULATION FILE/Subsystem5/Subsystem ==
  note: $I_{ph}=[I_{sc}+k_i.(T-298)].G/1000$
  T1 : Inport
  G1 : Inport  Port=2
  Add : Sum
  Constant : Constant  Value=298
  Constant1 : Constant  Value=ki
  Constant2 : Constant  Value=Isc1
  Constant3 : Constant  Value=1000
  Divide : Product  Inputs=*/
  Product : Product
  Product1 : Product
  Subtract : Sum  Inputs=+-
  Iph1 : Outport
  wires:
  G1/1 -> Product1/2
  Constant/1 -> Subtract/2
  T1/1 -> Subtract/1
  Subtract/1 -> Product/1
  Add/1 -> Product1/1
  Constant1/1 -> Product/2
  Product/1 -> Add/1
  Constant2/1 -> Add/2
  Product1/1 -> Divide/1
  Constant3/1 -> Divide/2
  Divide/1 -> Iph1/1

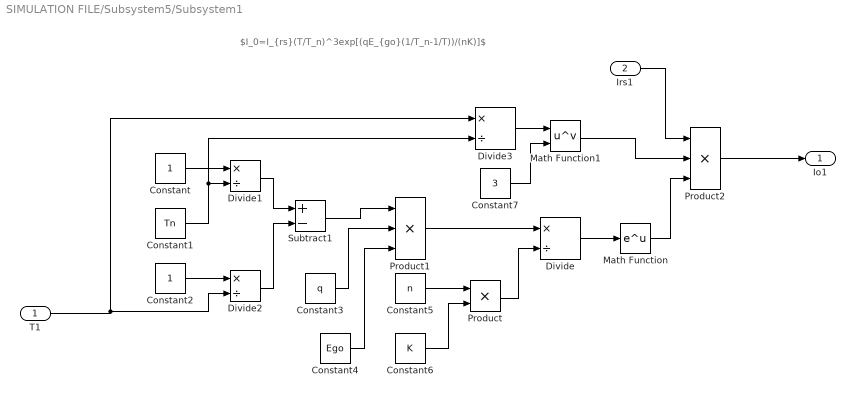
== system SIMULATION FILE/Subsystem5/Subsystem1 ==
  note: $I_0=I_{rs}(T/T_n)^3exp[(qE_{go}(1/T_n-1/T))/(nK)]$
  T1 : Inport
  Irs1 : Inport  Port=2
  Constant : Constant
  Constant1 : Constant  Value=Tn
  Constant2 : Constant
  Constant3 : Constant  Value=q
  Constant4 : Constant  Value=Ego
  Constant5 : Constant  Value=n
  Constant6 : Constant  Value=K
  Constant7 : Constant  Value=3
  Divide{,1..3} (4 alike) : Product  Inputs=*/
  Math Function : Math
  Math Function1 : Math  Operator=pow
  Product : Product
  Product1 : Product  Inputs=3
  Product2 : Product  Inputs=3
  Subtract1 : Sum  Inputs=+-
  Io1 : Outport
  wires:
  Constant6/1 -> Product/2
  Product1/1 -> Divide/1
  Math Function/1 -> Product2/3
  Subtract1/1 -> Product1/1
  Constant2/1 -> Divide2/1
  Divide3/1 -> Math Function1/1
  Divide/1 -> Math Function/1
  Constant7/1 -> Math Function1/2
  Irs1/1 -> Product2/1
  Product/1 -> Divide/2
  Divide1/1 -> Subtract1/1
  Constant5/1 -> Product/1
  Divide2/1 -> Subtract1/2
  T1/1 -> Divide3/1, Divide2/2
  Constant1/1 -> Divide3/2, Divide1/2
  Constant/1 -> Divide1/1
  Constant4/1 -> Product1/3
  Constant3/1 -> Product1/2
  Math Function1/1 -> Product2/2
  Product2/1 -> Io1/1

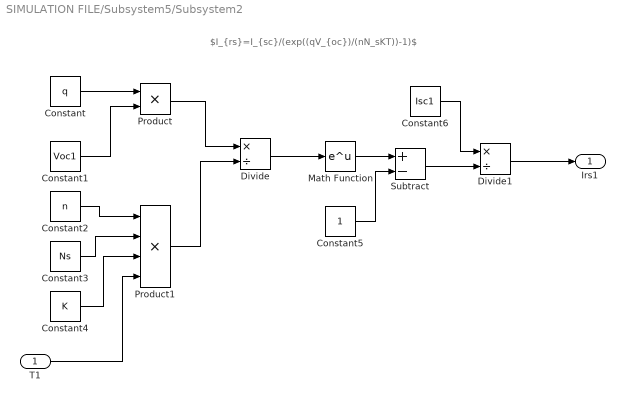
== system SIMULATION FILE/Subsystem5/Subsystem2 ==
  note: $I_{rs}=I_{sc}/(exp((qV_{oc})/(nN_sKT))-1)$
  T1 : Inport
  Constant : Constant  Value=q
  Constant1 : Constant  Value=Voc1
  Constant2 : Constant  Value=n
  Constant3 : Constant  Value=Ns
  Constant4 : Constant  Value=K
  Constant5 : Constant
  Constant6 : Constant  Value=Isc1
  Divide : Product  Inputs=*/
  Divide1 : Product  Inputs=*/
  Math Function : Math
  Product : Product
  Product1 : Product  Inputs=4
  Subtract : Sum  Inputs=+-
  Irs1 : Outport
  wires:
  Constant5/1 -> Subtract/2
  Product/1 -> Divide/1
  Subtract/1 -> Divide1/2
  Math Function/1 -> Subtract/1
  Divide1/1 -> Irs1/1
  Constant2/1 -> Product1/1
  Product1/1 -> Divide/2
  Constant1/1 -> Product/2
  Constant3/1 -> Product1/2
  Divide/1 -> Math Function/1
  Constant4/1 -> Product1/3
  Constant6/1 -> Divide1/1
  Constant/1 -> Product/1
  T1/1 -> Product1/4

== system SIMULATION FILE/Subsystem5/Subsystem3 ==
  note: $I_{sh}=(V+IR_{s})/R_{sh}$
  I1 : Inport
  V1 : Inport  Port=2
  Add : Sum
  Constant : Constant  Value=Rs1
  Constant1 : Constant  Value=Rsh1
  Divide : Product  Inputs=*/
  Product : Product
  Ish1 : Outport
  wires:
  Constant1/1 -> Divide/2
  Product/1 -> Add/1
  V1/1 -> Add/2
  I1/1 -> Product/2
  Divide/1 -> Ish1/1
  Constant/1 -> Product/1
  Add/1 -> Divide/1

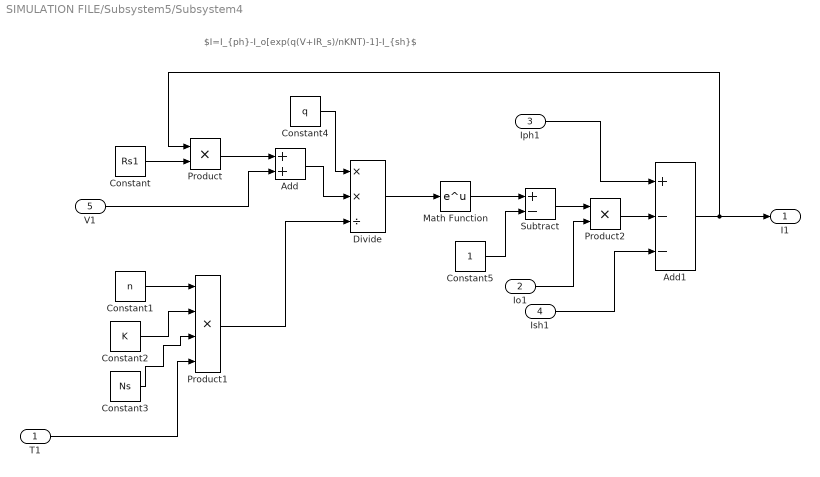
== system SIMULATION FILE/Subsystem5/Subsystem4 ==
  note: $I=I_{ph}-I_o[exp(q(V+IR_s)/nKNT)-1]-I_{sh}$
  T1 : Inport
  Io1 : Inport  Port=2
  Iph1 : Inport  Port=3
  Ish1 : Inport  Port=4
  V1 : Inport  Port=5
  Add : Sum
  Add1 : Sum  Inputs=+--
  Constant : Constant  Value=Rs1
  Constant1 : Constant  Value=n
  Constant2 : Constant  Value=K
  Constant3 : Constant  Value=Ns
  Constant4 : Constant  Value=q
  Constant5 : Constant
  Divide : Product  Inputs=**/
  Math Function : Math
  Product : Product
  Product1 : Product  Inputs=4
  Product2 : Product
  Subtract : Sum  Inputs=+-
  I1 : Outport
  wires:
  Constant3/1 -> Product1/3
  Subtract/1 -> Product2/1
  Constant1/1 -> Product1/1
  Divide/1 -> Math Function/1
  Constant4/1 -> Divide/1
  Product1/1 -> Divide/3
  Constant2/1 -> Product1/2
  Math Function/1 -> Subtract/1
  T1/1 -> Product1/4
  Product2/1 -> Add1/2
  Constant/1 -> Product/2
  Product/1 -> Add/1
  Constant5/1 -> Subtract/2
  Add/1 -> Divide/2
  Add1/1 -> I1/1, Product/1
  V1/1 -> Add/2
  Io1/1 -> Product2/2
  Ish1/1 -> Add1/3
  Iph1/1 -> Add1/1
